simulink model "EGR"  (R2020b)
settings: configuration reference "cs_ert" (kept outside this file)
settings Model: DataDictionary=EGR.sldd  EnableAccessToBaseWorkspace=off  Creator=zhoutinglin  LastModifiedBy=zhoutinglin
settings ConfigSetRef: SourceName=cs_ert

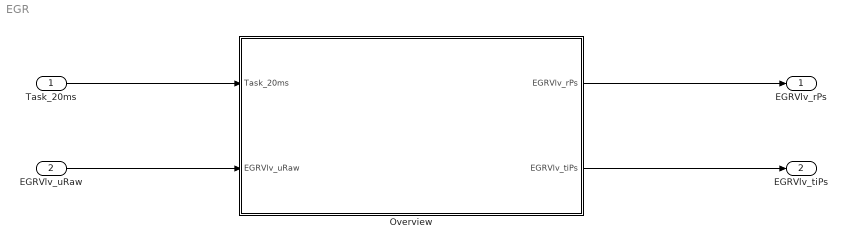
== system EGR ==
  Task_20ms : Inport  OutputFunctionCall=on
  EGRVlv_uRaw : Inport  Port=2
  Overview : Subsystem
  EGRVlv_rPs : Outport
  EGRVlv_tiPs : Outport  Port=2
  wires:
  Task_20ms/1 -> Overview/1(Task_20ms)
  EGRVlv_uRaw/1 -> Overview/2(EGRVlv_uRaw)
  Overview/1(EGRVlv_rPs) -> EGRVlv_rPs/1
  Overview/2(EGRVlv_tiPs) -> EGRVlv_tiPs/1

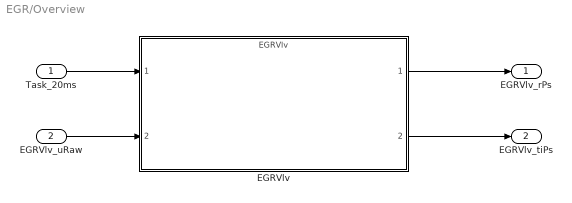
== system EGR/Overview ==
  Task_20ms : Inport
  EGRVlv_uRaw : Inport  Port=2
  EGRVlv : ModelReference  ModelNameDialog=EGRVlv  SimulationMode=Normal  ScheduleRates=on  ModelReferenceVersion=6.0
  EGRVlv_rPs : Outport
  EGRVlv_tiPs : Outport  Port=2
  wires:
  Task_20ms/1 -> EGRVlv/1
  EGRVlv_uRaw/1 -> EGRVlv/2
  EGRVlv/1 -> EGRVlv_rPs/1
  EGRVlv/2 -> EGRVlv_tiPs/1
